simulink model "SCARA_adaptive_passivity_controller"  (R2023b)
settings: Solver=VariableStepAuto  StartTime=0.0  StopTime=150  RelTol=1e-3
settings Model: Creator=Hamid Reza  LastModifiedBy=Hamid Reza

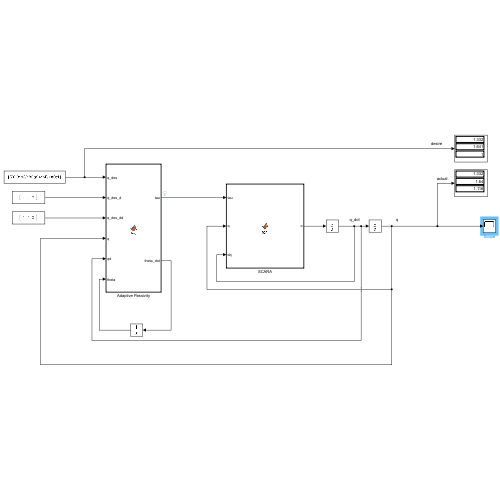
[thumbnail: Simulink's stored preview of the top-level diagram]
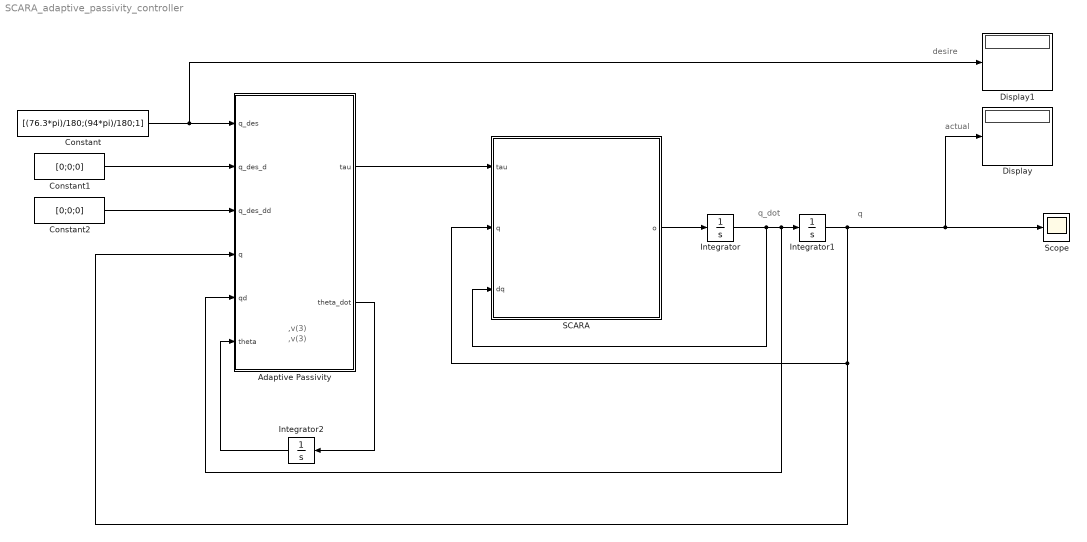
== system SCARA_adaptive_passivity_controller ==
  note: actual
  note: desire
  note: ,v(3)
  note: ,v(3)
  note: q_dot
  note: q
  Adaptive Passivity : MATLAB Function  TreatAsAtomicUnit=on
  Constant : Constant  Value=[(76.3*pi)/180;(94*pi)/180;1]
  Constant1 : Constant  Value=[0;0;0]
  Constant2 : Constant  Value=[0;0;0]
  Display : Display
  Display1 : Display
      settings: Decimation=3
  Integrator : Integrator  InitialCondition=[0;0;0]
  Integrator1 : Integrator  InitialCondition=[0;0;0]
  Integrator2 : Integrator
  SCARA : MATLAB Function  TreatAsAtomicUnit=on
  Scope : Scope
  wires:
  Integrator2/1 -> Adaptive Passivity/6(theta)
  Constant/1 -> Display1/1, Adaptive Passivity/1(q_des)
  Adaptive Passivity/2(theta_dot) -> Integrator2/1
  Constant2/1 -> Adaptive Passivity/3(q_des_dd)
  Adaptive Passivity/1(tau) -> SCARA/1(tau)
  Integrator/1 -> SCARA/3(dq), Adaptive Passivity/5(qd), Integrator1/1
  SCARA/1(o) -> Integrator/1
  Constant1/1 -> Adaptive Passivity/2(q_des_d)
  Integrator1/1 -> SCARA/2(q), Adaptive Passivity/4(q), Display/1, Scope/1

== matlab function SCARA_adaptive_passivity_controller/SCARA ==
  data: tau input; q input; dq input; o output
function o  = fcn(tau,q,dq)



theta1=q(1);
theta2=q(2);
d=q(3);

dtheta1=dq(1);
dtheta2=dq(2);
dd=dq(3);


a1=0.6;
a2=0.4;
m1=12;
m2=6;
m3=6;
g = 9.81;


% define mass matrix

m11 = (1/3)*m1*a1^2+m2*(a1^2+(1/3)*a2^2+a1*a2*cos(theta2))+m3*(a1^2+a2^2+2*a1*a2*cos(theta2));
m12 = -m2*a2*((1/3)*a2+(1/2)*a1*cos(theta2))-m3*(a2^2+a1*a2*cos(theta2));
m13 = 0;
m21 = m12;
m22 = (1/3)*m2*a2^2+m3*(a2^2);
m23 = 0;
m31 = m13;
m32 = m23;
m33 = m3;

M = [m11,m12,m13;m21,m22,m23;m31,m32,m33];


% define gravity matrix

g = [0; 0; -m3*g];

% define coriolis and centrifugal matrix

c1 = -(m2+2*m3)*a1*a2*sin(theta2)*(dtheta1*dtheta2+((1/2)*dtheta2^2));
c2 = ((1/2)*m2+m3)*a1*a2*sin(theta2)*(dtheta1^2);
c3 = 0;

C = [c1 ; c2 ; c3];


o=pinv(M)*(tau-(C+g));

== matlab function SCARA_adaptive_passivity_controller/Adaptive Passivity ==
  data: q_des input; q_des_d input; q_des_dd input; q input; qd input; tau output; theta_dot output; theta input
function [tau,theta_dot]= fcn(q_des,q_des_d,q_des_dd,q,qd,theta)
%%%%%%%%%%%%%%%%%%%%%%%%%%
q1=q(1);
q2=q(2);
d=q(3);


q1d=qd(1);
q2d=qd(2);
dd=qd(3);


%%%%%%%%%%
zita=1;
wn=2*pi*3;
K1=eye(3)*2*zita*wn;
K0=eye(3)*wn^2;
%%%%%%%%%%%
A=[zeros(3,3),eye(3);
    -K0,-K1];  
B=[zeros(3,3);eye(3)];

P=[  0.0664         0   -0.5000         0;
         0    0.0664         0   -0.5000;
   -0.5000         0    4.7257         0;
         0   -0.5000         0    4.7257];
%%%%%%%%
q_tilde=q-q_des;
q_tilde_d=qd-q_des_d;
e=[q_tilde;q_tilde_d];
%%%%%%%%%%%%%%%%%%%

q_tilde=q-q_des;
q_tilde_d=qd-q_des_d;

gamma=2;



v=q_des_d-gamma*q_tilde;
v_d=q_des_dd-gamma*q_tilde_d;
r=qd-v;

%important to see Y is function of v,vdot,q,qdot
Y1=[v_d(1),v_d(2),v(1)*q2d+v(2)*q1d+q2d*v(2),cos(q1),cos(q1+q2)];
Y2=[v_d(1),v_d(2),q1d*v(1),cos(q1+q2)];
Y3=[v(3)];

Y=blkdiag(Y1,Y2,Y3);

gam=.1;
theta_dot=-pinv(gam)*Y'*r;


K=5*eye(3);
tau=Y*theta-K*r;
